simulink model "mrefrobotarm_modified_previous_y_error_previous_u"  (R2018b)
settings: Solver=FixedStepAuto  StartTime=0.0  StopTime=60  RelTol=1e-3  AbsTol=1e-6
undefined symbols (not defined in the file or in its folder): now, sfunxy2, simin
libraries: neural x368, simulink x1
(part 6 of 10)

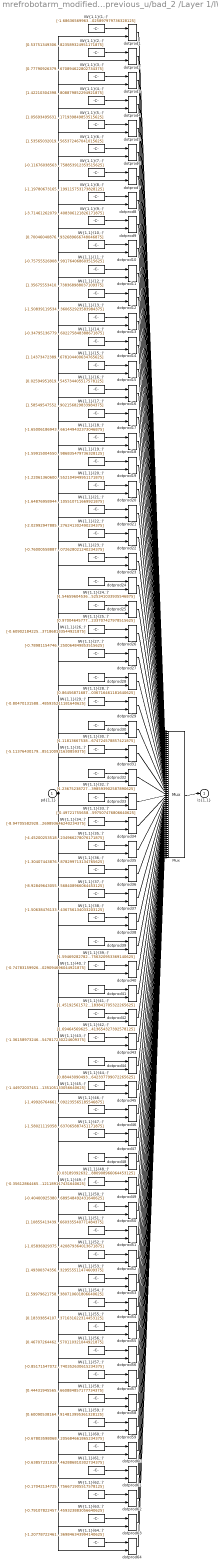
== system mrefrobotarm_modified_previous_y_error_previous_u/bad_2 /Layer 1/IW{1,1} ==
  "pd{1,1}" : Inport  PortDimensions=7
      mask Display: e = 0.06;c1 = [120 230 180]/255;c2 = ([120 230 180]+0)/(256+128);c3 = ([120 230 180]+128)/(256+128);patch([0 1 1 0],[0 0 1 1],c1);patch([0 1 1 1-e 1-e 0+e],[0 0 1 1-e 0+e 0+e],c2);patch([0 0 1 1-e 0+e 0+e],[0 1 1 1-e 1-e 0+e],c3);plot([0 1 1 0 0],[0 0 1 1 0]);
  "IW{1,1}(1,:)'" : Constant  Value=[-1.6863656996378744157283335880492813885211944580078125;-0.470597093744810790472143935403437353670597076416015625;0.381528307050592763172147670047706924378871917724609375;-1.12689962205123261895778341568075120449066162109375;-1.149898204806820256607124974834732711315155029296875;-1.0865193518723830212735492750653065741062164306640625;-0.6023983324376900316821092928876169025897979736328125]
      mask Display: e = 0.06;c1 = [120 150 230]/255;c2 = ([120 150 230]+0)/383;c3 = ([120 150 230]+128)/383;patch([0 1 1 0],[0 0 1 1],c1);patch([0 1 1 1-e 1-e 0+e],[0 0 1 1-e 0+e 0+e],c2);patch([0 0 1 1-e 0+e 0+e],[0 1 1 1-e 1-e 0+e],c3);plot([0 1 1 0 0],[0 0 1 1 0]);disp('Weights');
  "IW{1,1}(10,:)'" : Constant  Value=[0.70046040876794501972568696146481670439243316650390625;-0.59634747279149558085720173039590008556842803955078125;0.33402845316572282730049892052193172276020050048828125;-0.1546411702019059308810255970456637442111968994140625;1.35413836861219305518488909001462161540985107421875;1.7346283899615413393036078559816814959049224853515625;-0.56975117430301647214463400814565829932689666748046875]
      mask Display: e = 0.06;c1 = [120 150 230]/255;c2 = ([120 150 230]+0)/383;c3 = ([120 150 230]+128)/383;patch([0 1 1 0],[0 0 1 1],c1);patch([0 1 1 1-e 1-e 0+e],[0 0 1 1-e 0+e 0+e],c2);patch([0 0 1 1-e 0+e 0+e],[0 1 1 1-e 1-e 0+e],c3);plot([0 1 1 0 0],[0 0 1 1 0]);disp('Weights');
  "IW{1,1}(11,:)'" : Constant  Value=[-0.75755526908276149544718691686284728348255157470703125;-0.296579563589438433002243300506961531937122344970703125;0.497779535965763575422471376441535539925098419189453125;0.1665504115849312238850643552723340690135955810546875;-1.643932170348186172503801572020165622234344482421875;0.8794875708418334880889233318157494068145751953125;1.1526104705362014701819362016976810991764068603515625]
      mask Display: e = 0.06;c1 = [120 150 230]/255;c2 = ([120 150 230]+0)/383;c3 = ([120 150 230]+128)/383;patch([0 1 1 0],[0 0 1 1],c1);patch([0 1 1 1-e 1-e 0+e],[0 0 1 1-e 0+e 0+e],c2);patch([0 0 1 1-e 0+e 0+e],[0 1 1 1-e 1-e 0+e],c3);plot([0 1 1 0 0],[0 0 1 1 0]);disp('Weights');
  "IW{1,1}(12,:)'" : Constant  Value=[1.356755534102476179469931594212539494037628173828125;0.8249762999779475247663640402606688439846038818359375;0.11116932047618825751822413394620525650680065155029296875;-0.40444127320000544667522035524598322808742523193359375;-0.7395790815915237459421405219472944736480712890625;-1.102233156945345182720075172255747020244598388671875;1.5180689591781619807164815938449464738368988037109375]
      mask Display: e = 0.06;c1 = [120 150 230]/255;c2 = ([120 150 230]+0)/383;c3 = ([120 150 230]+128)/383;patch([0 1 1 0],[0 0 1 1],c1);patch([0 1 1 1-e 1-e 0+e],[0 0 1 1-e 0+e 0+e],c2);patch([0 0 1 1-e 0+e 0+e],[0 1 1 1-e 1-e 0+e],c3);plot([0 1 1 0 0],[0 0 1 1 0]);disp('Weights');
  "IW{1,1}(13,:)'" : Constant  Value=[-1.508391195342500878950886544771492481231689453125;0.1745384352813305894880357982401619665324687957763671875;-0.35046267193310509657777629399788565933704376220703125;0.70755991279883534428307712005334906280040740966796875;0.21164846614004406699649507572758011519908905029296875;3.394560192280937638287241497891955077648162841796875;2.8592038307015368303609648137353360652923583984375]
      mask Display: e = 0.06;c1 = [120 150 230]/255;c2 = ([120 150 230]+0)/383;c3 = ([120 150 230]+128)/383;patch([0 1 1 0],[0 0 1 1],c1);patch([0 1 1 1-e 1-e 0+e],[0 0 1 1-e 0+e 0+e],c2);patch([0 0 1 1-e 0+e 0+e],[0 1 1 1-e 1-e 0+e],c3);plot([0 1 1 0 0],[0 0 1 1 0]);disp('Weights');
  "IW{1,1}(14,:)'" : Constant  Value=[-0.347951367798633726113877173702348954975605010986328125;-1.1758278102151298316613292627152986824512481689453125;-1.4111353580198293666825293257716111838817596435546875;0.452708396797978529502159972253139130771160125732421875;0.57952339232880223374166916983085684478282928466796875;1.5762379928547864960108881859923712909221649169921875;0.9810342317283140545214337180368602275848388671875]
      mask Display: e = 0.06;c1 = [120 150 230]/255;c2 = ([120 150 230]+0)/383;c3 = ([120 150 230]+128)/383;patch([0 1 1 0],[0 0 1 1],c1);patch([0 1 1 1-e 1-e 0+e],[0 0 1 1-e 0+e 0+e],c2);patch([0 0 1 1-e 0+e 0+e],[0 1 1 1-e 1-e 0+e],c3);plot([0 1 1 0 0],[0 0 1 1 0]);disp('Weights');
  "IW{1,1}(15,:)'" : Constant  Value=[1.14373472389301156226792954839766025543212890625;0.9770289905242410810615183436311781406402587890625;-0.918973607377620016478658726555295288562774658203125;0.872028597290672724540172566776163876056671142578125;1.4709013012625096195051810354925692081451416015625;-0.1290434951660533735573466174173518083989620208740234375;0.66656798656280236148319318090216256678104400634765625]
      mask Display: e = 0.06;c1 = [120 150 230]/255;c2 = ([120 150 230]+0)/383;c3 = ([120 150 230]+128)/383;patch([0 1 1 0],[0 0 1 1],c1);patch([0 1 1 1-e 1-e 0+e],[0 0 1 1-e 0+e 0+e],c2);patch([0 0 1 1-e 0+e 0+e],[0 1 1 1-e 1-e 0+e],c3);plot([0 1 1 0 0],[0 0 1 1 0]);disp('Weights');
  "IW{1,1}(16,:)'" : Constant  Value=[0.025949518194994046493828676602788618765771389007568359375;1.056286903314246128360309739946387708187103271484375;1.3864161845839706455052464662003330886363983154296875;-0.62378102653036349156678852523327805101871490478515625;2.046193686105493458882165214163251221179962158203125;-0.0948604936613626492647455279438872821629047393798828125;1.4769159957528821269789887082879431545734405517578125]
      mask Display: e = 0.06;c1 = [120 150 230]/255;c2 = ([120 150 230]+0)/383;c3 = ([120 150 230]+128)/383;patch([0 1 1 0],[0 0 1 1],c1);patch([0 1 1 1-e 1-e 0+e],[0 0 1 1-e 0+e 0+e],c2);patch([0 0 1 1-e 0+e 0+e],[0 1 1 1-e 1-e 0+e],c3);plot([0 1 1 0 0],[0 0 1 1 0]);disp('Weights');
  "IW{1,1}(17,:)'" : Constant  Value=[1.5854954755240395769533279235474765300750732421875;0.062584963321976549988079341346747241914272308349609375;-1.086219183721052861102407405269332230091094970703125;-0.472400812961043137239158795637194998562335968017578125;-0.2084756610371170937323626048964797519147396087646484375;-1.2682346351539524054174989942112006247043609619140625;-2.59195409337992455078847342520020902156829833984375]
      mask Display: e = 0.06;c1 = [120 150 230]/255;c2 = ([120 150 230]+0)/383;c3 = ([120 150 230]+128)/383;patch([0 1 1 0],[0 0 1 1],c1);patch([0 1 1 1-e 1-e 0+e],[0 0 1 1-e 0+e 0+e],c2);patch([0 0 1 1-e 0+e 0+e],[0 1 1 1-e 1-e 0+e],c3);plot([0 1 1 0 0],[0 0 1 1 0]);disp('Weights');
  "IW{1,1}(18,:)'" : Constant  Value=[-1.6500618694364199701141160403494723141193389892578125;0.158471949334514750074021094405907206237316131591796875;1.605402587803847591629846647265367209911346435546875;-0.3344369037299077529468149805325083434581756591796875;0.357965741888847055474087710535968653857707977294921875;-2.016135923701856125234144201385788619518280029296875;-0.460005488291919728549572710107895545661449432373046875]
      mask Display: e = 0.06;c1 = [120 150 230]/255;c2 = ([120 150 230]+0)/383;c3 = ([120 150 230]+128)/383;patch([0 1 1 0],[0 0 1 1],c1);patch([0 1 1 1-e 1-e 0+e],[0 0 1 1-e 0+e 0+e],c2);patch([0 0 1 1-e 0+e 0+e],[0 1 1 1-e 1-e 0+e],c3);plot([0 1 1 0 0],[0 0 1 1 0]);disp('Weights');
  "IW{1,1}(19,:)'" : Constant  Value=[-1.5991500455075655651171473436988890171051025390625;1.348245600949198763629510722239501774311065673828125;0.80807469706489853944475498792598955333232879638671875;-1.7624762240675149183033454391988925635814666748046875;-1.016806479705910870592333594686351716518402099609375;0.300813059873307808711473398943780921399593353271484375;-1.634726680080462291044796074857003986835479736328125]
      mask Display: e = 0.06;c1 = [120 150 230]/255;c2 = ([120 150 230]+0)/383;c3 = ([120 150 230]+128)/383;patch([0 1 1 0],[0 0 1 1],c1);patch([0 1 1 1-e 1-e 0+e],[0 0 1 1-e 0+e 0+e],c2);patch([0 0 1 1-e 0+e 0+e],[0 1 1 1-e 1-e 0+e],c3);plot([0 1 1 0 0],[0 0 1 1 0]);disp('Weights');
  "IW{1,1}(2,:)'" : Constant  Value=[0.5375134930612259775983829968026839196681976318359375;-0.24811864763972335534703006487688980996608734130859375;-0.9050550568703263909497991335229016840457916259765625;-1.330177669034877663278848558547906577587127685546875;0.8445151037025706575178674029302783310413360595703125;0.453823539254982255553017012061900459229946136474609375;1.51432188940290313183822945575229823589324951171875]
      mask Display: e = 0.06;c1 = [120 150 230]/255;c2 = ([120 150 230]+0)/383;c3 = ([120 150 230]+128)/383;patch([0 1 1 0],[0 0 1 1],c1);patch([0 1 1 1-e 1-e 0+e],[0 0 1 1-e 0+e 0+e],c2);patch([0 0 1 1-e 0+e 0+e],[0 1 1 1-e 1-e 0+e],c3);plot([0 1 1 0 0],[0 0 1 1 0]);disp('Weights');
  "IW{1,1}(20,:)'" : Constant  Value=[-1.2206136060051242520074765707249753177165985107421875;1.2143694024926621199966803033021278679370880126953125;0.01284061424074450959154081175483952392823994159698486328125;0.674556463178389353885222590179182589054107666015625;0.82271266002563281372061965157627128064632415771484375;1.4603421023320530824918250800692476332187652587890625;-1.023340866984355113089577571372501552104949951171875]
      mask Display: e = 0.06;c1 = [120 150 230]/255;c2 = ([120 150 230]+0)/383;c3 = ([120 150 230]+128)/383;patch([0 1 1 0],[0 0 1 1],c1);patch([0 1 1 1-e 1-e 0+e],[0 0 1 1-e 0+e 0+e],c2);patch([0 0 1 1-e 0+e 0+e],[0 1 1 1-e 1-e 0+e],c3);plot([0 1 1 0 0],[0 0 1 1 0]);disp('Weights');
  "IW{1,1}(21,:)'" : Constant  Value=[-1.648769589442328875605880966759286820888519287109375;0.5674233186469184175848567974753677845001220703125;0.360630049005453423571765370070352219045162200927734375;0.72618846736561659671593815801315940916538238525390625;-1.6863477747584882937559314086684025824069976806640625;-0.543238509671011282620156634948216378688812255859375;-0.82507519282673491556323597251321189105510711669921875]
      mask Display: e = 0.06;c1 = [120 150 230]/255;c2 = ([120 150 230]+0)/383;c3 = ([120 150 230]+128)/383;patch([0 1 1 0],[0 0 1 1],c1);patch([0 1 1 1-e 1-e 0+e],[0 0 1 1-e 0+e 0+e],c2);patch([0 0 1 1-e 0+e 0+e],[0 1 1 1-e 1-e 0+e],c3);plot([0 1 1 0 0],[0 0 1 1 0]);disp('Weights');
  "IW{1,1}(22,:)'" : Constant  Value=[-2.02992947885647989636481725028716027736663818359375;-0.78930300349707904761231702650547958910465240478515625;-1.600745458741919424738853194867260754108428955078125;2.151514262201442040378651654464192688465118408203125;1.4383445102898109180245000970899127423763275146484375;1.0715968603907735090530195520841516554355621337890625;0.29850111989870364848087547215982340276241302490234375]
      mask Display: e = 0.06;c1 = [120 150 230]/255;c2 = ([120 150 230]+0)/383;c3 = ([120 150 230]+128)/383;patch([0 1 1 0],[0 0 1 1],c1);patch([0 1 1 1-e 1-e 0+e],[0 0 1 1-e 0+e 0+e],c2);patch([0 0 1 1-e 0+e 0+e],[0 1 1 1-e 1-e 0+e],c3);plot([0 1 1 0 0],[0 0 1 1 0]);disp('Weights');
  "IW{1,1}(23,:)'" : Constant  Value=[-0.7600055888729659869795796112157404422760009765625;0.71322247233798297116891262703575193881988525390625;1.917261913113857740853518407675437629222869873046875;0.056807101221510995781027730799905839376151561737060546875;0.6989265569105611586309123595128767192363739013671875;2.165339178672456288410330671467818319797515869140625;0.274757432287420166883151750880642794072628021240234375]
      mask Display: e = 0.06;c1 = [120 150 230]/255;c2 = ([120 150 230]+0)/383;c3 = ([120 150 230]+128)/383;patch([0 1 1 0],[0 0 1 1],c1);patch([0 1 1 1-e 1-e 0+e],[0 0 1 1-e 0+e 0+e],c2);patch([0 0 1 1-e 0+e 0+e],[0 1 1 1-e 1-e 0+e],c3);plot([0 1 1 0 0],[0 0 1 1 0]);disp('Weights');
  "IW{1,1}(24,:)'" : Constant  Value=[1.546596045364299509827787915128283202648162841796875;-1.8043253491178485869994574386510066688060760498046875;-1.0873028546852918641008045597118325531482696533203125;0.489548897640237345996183648821897804737091064453125;-1.0685662650111333871194574385299347341060638427734375;-2.01145955325918013301134124048985540866851806640625;-1.086944648018185244353617235901765525341033935546875]
      mask Display: e = 0.06;c1 = [120 150 230]/255;c2 = ([120 150 230]+0)/383;c3 = ([120 150 230]+128)/383;patch([0 1 1 0],[0 0 1 1],c1);patch([0 1 1 1-e 1-e 0+e],[0 0 1 1-e 0+e 0+e],c2);patch([0 0 1 1-e 0+e 0+e],[0 1 1 1-e 1-e 0+e],c3);plot([0 1 1 0 0],[0 0 1 1 0]);disp('Weights');
  "IW{1,1}(25,:)'" : Constant  Value=[0.97004645777546294471704868556116707623004913330078125;0.336271611140263881889467256769421510398387908935546875;0.2417062721643864764420328583582886494696140289306640625;1.4989475360339128418019072341849096119403839111328125;1.4380511250646048626578021867317147552967071533203125;1.1249383286835179518448057933710515499114990234375;0.2251758799012057166155642562443972565233707427978515625]
      mask Display: e = 0.06;c1 = [120 150 230]/255;c2 = ([120 150 230]+0)/383;c3 = ([120 150 230]+128)/383;patch([0 1 1 0],[0 0 1 1],c1);patch([0 1 1 1-e 1-e 0+e],[0 0 1 1-e 0+e 0+e],c2);patch([0 0 1 1-e 0+e 0+e],[0 1 1 1-e 1-e 0+e],c3);plot([0 1 1 0 0],[0 0 1 1 0]);disp('Weights');
  "IW{1,1}(26,:)'" : Constant  Value=[-0.60902184225669453443430256811552681028842926025390625;1.4626237168885207751145571819506585597991943359375;-0.283646747149560118916866713334457017481327056884765625;-0.41578668224785364504469953317311592400074005126953125;1.8146939194076010526401887545944191515445709228515625;-0.94831384411612063001228989378432743251323699951171875;0.99177285614588306383865301540936343371868133544921875]
      mask Display: e = 0.06;c1 = [120 150 230]/255;c2 = ([120 150 230]+0)/383;c3 = ([120 150 230]+128)/383;patch([0 1 1 0],[0 0 1 1],c1);patch([0 1 1 1-e 1-e 0+e],[0 0 1 1-e 0+e 0+e],c2);patch([0 0 1 1-e 0+e 0+e],[0 1 1 1-e 1-e 0+e],c3);plot([0 1 1 0 0],[0 0 1 1 0]);disp('Weights');
  "IW{1,1}(27,:)'" : Constant  Value=[-0.78981154746552861833919223499833606183528900146484375;-1.3508127899859114773306600909563712775707244873046875;0.4988288733380119577276445852476172149181365966796875;-0.761291513497599492410472521441988646984100341796875;1.513839332845589691345367100439034402370452880859375;1.038568147474759228998664184473454952239990234375;-1.2619104742456475065637278021313250064849853515625]
      mask Display: e = 0.06;c1 = [120 150 230]/255;c2 = ([120 150 230]+0)/383;c3 = ([120 150 230]+128)/383;patch([0 1 1 0],[0 0 1 1],c1);patch([0 1 1 1-e 1-e 0+e],[0 0 1 1-e 0+e 0+e],c2);patch([0 0 1 1-e 0+e 0+e],[0 1 1 1-e 1-e 0+e],c3);plot([0 1 1 0 0],[0 0 1 1 0]);disp('Weights');
  "IW{1,1}(28,:)'" : Constant  Value=[0.86456871687262815129315640660934150218963623046875;0.033660231342696848855222668817077646963298320770263671875;0.68849562687325371879154545240453444421291351318359375;1.05512528935876037650132275302894413471221923828125;1.3310343837191738192160528342355974018573760986328125;1.4214566142145310667643798296921886503696441650390625;-0.91698163671545673825136191226192750036716461181640625]
      mask Display: e = 0.06;c1 = [120 150 230]/255;c2 = ([120 150 230]+0)/383;c3 = ([120 150 230]+128)/383;patch([0 1 1 0],[0 0 1 1],c1);patch([0 1 1 1-e 1-e 0+e],[0 0 1 1-e 0+e 0+e],c2);patch([0 0 1 1-e 0+e 0+e],[0 1 1 1-e 1-e 0+e],c3);plot([0 1 1 0 0],[0 0 1 1 0]);disp('Weights');
  "IW{1,1}(29,:)'" : Constant  Value=[-0.80470131588495730223797863800427876412868499755859375;-1.6155846603753911683298838397604413330554962158203125;-0.29114476463801874928094548522494733333587646484375;0.75042474844354678520375045991386286914348602294921875;1.7495307116501146449394354931428097188472747802734375;-0.3413257555915460983442244469188153743743896484375;-0.382665686428625806403402975774952210485935211181640625]
      mask Display: e = 0.06;c1 = [120 150 230]/255;c2 = ([120 150 230]+0)/383;c3 = ([120 150 230]+128)/383;patch([0 1 1 0],[0 0 1 1],c1);patch([0 1 1 1-e 1-e 0+e],[0 0 1 1-e 0+e 0+e],c2);patch([0 0 1 1-e 0+e 0+e],[0 1 1 1-e 1-e 0+e],c3);plot([0 1 1 0 0],[0 0 1 1 0]);disp('Weights');
  "IW{1,1}(3,:)'" : Constant  Value=[0.77790926379179115013329237626749090850353240966796875;1.597997887025701668761712426203303039073944091796875;-0.061513463120482343715611506240747985430061817169189453125;0.7694262824388911070627727895043790340423583984375;0.53571795086796225593417375421267934143543243408203125;1.255108578389512619111201274790801107883453369140625;-1.12287357758761885406784131191670894622802734375]
      mask Display: e = 0.06;c1 = [120 150 230]/255;c2 = ([120 150 230]+0)/383;c3 = ([120 150 230]+128)/383;patch([0 1 1 0],[0 0 1 1],c1);patch([0 1 1 1-e 1-e 0+e],[0 0 1 1-e 0+e 0+e],c2);patch([0 0 1 1-e 0+e 0+e],[0 1 1 1-e 1-e 0+e],c3);plot([0 1 1 0 0],[0 0 1 1 0]);disp('Weights');
  "IW{1,1}(30,:)'" : Constant  Value=[1.11813667538101402243455595453269779682159423828125;-2.0011147436250649178646199288778007030487060546875;-1.2389603095632202300890867263660766184329986572265625;0.99632266524748314129311665965360589325428009033203125;-0.1464403285517131558801651181056513451039791107177734375;1.78125755432936383471087538055144250392913818359375;1.7380547403563877395527015323750674724578857421875]
      mask Display: e = 0.06;c1 = [120 150 230]/255;c2 = ([120 150 230]+0)/383;c3 = ([120 150 230]+128)/383;patch([0 1 1 0],[0 0 1 1],c1);patch([0 1 1 1-e 1-e 0+e],[0 0 1 1-e 0+e 0+e],c2);patch([0 0 1 1-e 0+e 0+e],[0 1 1 1-e 1-e 0+e],c3);plot([0 1 1 0 0],[0 0 1 1 0]);disp('Weights');
  "IW{1,1}(31,:)'" : Constant  Value=[-5.1137643017961860181230804300867021083831787109375;1.3370606083956821930058822545106522738933563232421875;2.442518793233874330184107748209498822689056396484375;0.6028625806456482383310913064633496105670928955078125;-1.92576905446539026200980515568517148494720458984375;-0.6757333917518464350138174268067814409732818603515625;0.81038330323658624987359644364914856851100921630859375]
      mask Display: e = 0.06;c1 = [120 150 230]/255;c2 = ([120 150 230]+0)/383;c3 = ([120 150 230]+128)/383;patch([0 1 1 0],[0 0 1 1],c1);patch([0 1 1 1-e 1-e 0+e],[0 0 1 1-e 0+e 0+e],c2);patch([0 0 1 1-e 0+e 0+e],[0 1 1 1-e 1-e 0+e],c3);plot([0 1 1 0 0],[0 0 1 1 0]);disp('Weights');
  "IW{1,1}(32,:)'" : Constant  Value=[1.2367523872787222760649683550582267343997955322265625;-0.784854563913853997547676044632680714130401611328125;-1.439473545848857671813902925350703299045562744140625;1.09236546200067241585429655970074236392974853515625;1.0496288292411153353356212392100133001804351806640625;0.06836094254987955254332376853199093602597713470458984375;-1.286462130941723902566309334360994398593902587890625]
      mask Display: e = 0.06;c1 = [120 150 230]/255;c2 = ([120 150 230]+0)/383;c3 = ([120 150 230]+128)/383;patch([0 1 1 0],[0 0 1 1],c1);patch([0 1 1 1-e 1-e 0+e],[0 0 1 1-e 0+e 0+e],c2);patch([0 0 1 1-e 0+e 0+e],[0 1 1 1-e 1-e 0+e],c3);plot([0 1 1 0 0],[0 0 1 1 0]);disp('Weights');
  "IW{1,1}(33,:)'" : Constant  Value=[-0.4972175565835499355671345256268978118896484375;1.01628497643774817760231599095277488231658935546875;1.705775427614244943441690338659100234508514404296875;-0.155163647387632275265190173740847967565059661865234375;-0.38711282558761184180440295676817186176776885986328125;0.6706206203731606141360543915652669966220855712890625;-1.11530850752759480570830419310368597507476806640625]
      mask Display: e = 0.06;c1 = [120 150 230]/255;c2 = ([120 150 230]+0)/383;c3 = ([120 150 230]+128)/383;patch([0 1 1 0],[0 0 1 1],c1);patch([0 1 1 1-e 1-e 0+e],[0 0 1 1-e 0+e 0+e],c2);patch([0 0 1 1-e 0+e 0+e],[0 1 1 1-e 1-e 0+e],c3);plot([0 1 1 0 0],[0 0 1 1 0]);disp('Weights');
  "IW{1,1}(34,:)'" : Constant  Value=[-8.9470558292806234845784274511970579624176025390625;5.86025071287466925440412524039857089519500732421875;0.89003059289749819615877868272946216166019439697265625;-0.006319623623432799215671185066867110435850918292999267578125;1.1887800724449284484052213883842341601848602294921875;3.9517133987949062401412447798065841197967529296875;2.4410282631594579783040899201296269893646240234375]
      mask Display: e = 0.06;c1 = [120 150 230]/255;c2 = ([120 150 230]+0)/383;c3 = ([120 150 230]+128)/383;patch([0 1 1 0],[0 0 1 1],c1);patch([0 1 1 1-e 1-e 0+e],[0 0 1 1-e 0+e 0+e],c2);patch([0 0 1 1-e 0+e 0+e],[0 1 1 1-e 1-e 0+e],c3);plot([0 1 1 0 0],[0 0 1 1 0]);disp('Weights');
  "IW{1,1}(35,:)'" : Constant  Value=[-4.45200253518322863754974605399183928966522216796875;1.0956730899398532397270855653914622962474822998046875;-0.296116424887555407252648365101777017116546630859375;1.494172243435615943241145942010916769504547119140625;-1.405105462929962190088417628430761396884918212890625;-1.8065586582246557778574924668646417558193206787109375;-2.091504311274504868123358392040245234966278076171875]
      mask Display: e = 0.06;c1 = [120 150 230]/255;c2 = ([120 150 230]+0)/383;c3 = ([120 150 230]+128)/383;patch([0 1 1 0],[0 0 1 1],c1);patch([0 1 1 1-e 1-e 0+e],[0 0 1 1-e 0+e 0+e],c2);patch([0 0 1 1-e 0+e 0+e],[0 1 1 1-e 1-e 0+e],c3);plot([0 1 1 0 0],[0 0 1 1 0]);disp('Weights');
  "IW{1,1}(36,:)'" : Constant  Value=[-1.3040744387684621852230293370666913688182830810546875;-1.0839533773058225296637147039291448891162872314453125;1.1996912135972817026186021394096314907073974609375;0.299632799474621902557913699638447724282741546630859375;-1.0338437717971202811639841456781141459941864013671875;1.060633860379795123662916012108325958251953125;0.80119404908470548409837874714867211878299713134765625]
      mask Display: e = 0.06;c1 = [120 150 230]/255;c2 = ([120 150 230]+0)/383;c3 = ([120 150 230]+128)/383;patch([0 1 1 0],[0 0 1 1],c1);patch([0 1 1 1-e 1-e 0+e],[0 0 1 1-e 0+e 0+e],c2);patch([0 0 1 1-e 0+e 0+e],[0 1 1 1-e 1-e 0+e],c3);plot([0 1 1 0 0],[0 0 1 1 0]);disp('Weights');
  "IW{1,1}(37,:)'" : Constant  Value=[-8.928496430556503327125028590671718120574951171875;6.41281098021677653520100648165680468082427978515625;1.292318686852158560185444002854637801647186279296875;-1.0169657309557076363404348740004934370517730712890625;-1.4447233934709735603263425218756310641765594482421875;-1.8212597060116382241545807119109667837619781494140625;-2.000066902793254275394474461791105568408966064453125]
      mask Display: e = 0.06;c1 = [120 150 230]/255;c2 = ([120 150 230]+0)/383;c3 = ([120 150 230]+128)/383;patch([0 1 1 0],[0 0 1 1],c1);patch([0 1 1 1-e 1-e 0+e],[0 0 1 1-e 0+e 0+e],c2);patch([0 0 1 1-e 0+e 0+e],[0 1 1 1-e 1-e 0+e],c3);plot([0 1 1 0 0],[0 0 1 1 0]);disp('Weights');
  "IW{1,1}(38,:)'" : Constant  Value=[-1.5063847613337173481085073944996111094951629638671875;-0.92097648878295623742218367624445818364620208740234375;-0.9838165288434570499020992428995668888092041015625;-0.33928758212320830889296985333203338086605072021484375;-0.60176867956408575111026948434300720691680908203125;0.52167233477996066692838894596206955611705780029296875;-0.901664409713287984260432494920678436756134033203125]
      mask Display: e = 0.06;c1 = [120 150 230]/255;c2 = ([120 150 230]+0)/383;c3 = ([120 150 230]+128)/383;patch([0 1 1 0],[0 0 1 1],c1);patch([0 1 1 1-e 1-e 0+e],[0 0 1 1-e 0+e 0+e],c2);patch([0 0 1 1-e 0+e 0+e],[0 1 1 1-e 1-e 0+e],c3);plot([0 1 1 0 0],[0 0 1 1 0]);disp('Weights');
  "IW{1,1}(39,:)'" : Constant  Value=[1.594692827829733428046665721922181546688079833984375;-0.431588743177177491805451836626161821186542510986328125;-0.5767038172813823138085354003123939037322998046875;-1.4856881211963273159426535130478441715240478515625;-1.537250986312717504489455677685327827930450439453125;-1.5160546591084627099377257763990201056003570556640625;0.02677171951358392476549852290190756320953369140625]
      mask Display: e = 0.06;c1 = [120 150 230]/255;c2 = ([120 150 230]+0)/383;c3 = ([120 150 230]+128)/383;patch([0 1 1 0],[0 0 1 1],c1);patch([0 1 1 1-e 1-e 0+e],[0 0 1 1-e 0+e 0+e],c2);patch([0 0 1 1-e 0+e 0+e],[0 1 1 1-e 1-e 0+e],c3);plot([0 1 1 0 0],[0 0 1 1 0]);disp('Weights');
  "IW{1,1}(4,:)'" : Constant  Value=[1.4221030439802160305617917401832528412342071533203125;-0.719802079075858358692130423150956630706787109375;0.390203414206296839150667210560641251504421234130859375;-1.40290775448764382105082404450513422489166259765625;-0.246566272133671715582892147722304798662662506103515625;0.978533484262781971807498848647810518741607666015625;0.72315047260570686216141211843932978808879852294921875]
      mask Display: e = 0.06;c1 = [120 150 230]/255;c2 = ([120 150 230]+0)/383;c3 = ([120 150 230]+128)/383;patch([0 1 1 0],[0 0 1 1],c1);patch([0 1 1 1-e 1-e 0+e],[0 0 1 1-e 0+e 0+e],c2);patch([0 0 1 1-e 0+e 0+e],[0 1 1 1-e 1-e 0+e],c3);plot([0 1 1 0 0],[0 0 1 1 0]);disp('Weights');
  "IW{1,1}(40,:)'" : Constant  Value=[-0.74783159926091802294223498392966575920581817626953125;-0.0156016786915698472959501685863870079629123210906982421875;1.205674453621349950793728567077778279781341552734375;-0.642379166939826884430431164219044148921966552734375;-2.3466396920997372177453144104219973087310791015625;2.003758055175307806194950899225659668445587158203125;0.457948677082519572945074060044134967029094696044921875]
      mask Display: e = 0.06;c1 = [120 150 230]/255;c2 = ([120 150 230]+0)/383;c3 = ([120 150 230]+128)/383;patch([0 1 1 0],[0 0 1 1],c1);patch([0 1 1 1-e 1-e 0+e],[0 0 1 1-e 0+e 0+e],c2);patch([0 0 1 1-e 0+e 0+e],[0 1 1 1-e 1-e 0+e],c3);plot([0 1 1 0 0],[0 0 1 1 0]);disp('Weights');
  "IW{1,1}(41,:)'" : Constant  Value=[1.451925615721403328706173851969651877880096435546875;0.893887593572912475536895726691000163555145263671875;-0.47449044571051024465901946314261294901371002197265625;-1.1508731751823262356992927379906177520751953125;-0.45410349609860478636846892186440527439117431640625;0.194166359333692917221725338094984181225299835205078125;-1.4499390721543312654517876580939628183841705322265625]
      mask Display: e = 0.06;c1 = [120 150 230]/255;c2 = ([120 150 230]+0)/383;c3 = ([120 150 230]+128)/383;patch([0 1 1 0],[0 0 1 1],c1);patch([0 1 1 1-e 1-e 0+e],[0 0 1 1-e 0+e 0+e],c2);patch([0 0 1 1-e 0+e 0+e],[0 1 1 1-e 1-e 0+e],c3);plot([0 1 1 0 0],[0 0 1 1 0]);disp('Weights');
  "IW{1,1}(42,:)'" : Constant  Value=[1.6946456962588474226549806189723312854766845703125;0.425834425212213874001321300966083072125911712646484375;-0.12820727712798618558309726722654886543750762939453125;0.82693407426810916494019920719438232481479644775390625;-0.686592815915464171894200262613594532012939453125;-1.758457794378568639359627923113293945789337158203125;-1.16195091792224758364682202227413654327392578125]
      mask Display: e = 0.06;c1 = [120 150 230]/255;c2 = ([120 150 230]+0)/383;c3 = ([120 150 230]+128)/383;patch([0 1 1 0],[0 0 1 1],c1);patch([0 1 1 1-e 1-e 0+e],[0 0 1 1-e 0+e 0+e],c2);patch([0 0 1 1-e 0+e 0+e],[0 1 1 1-e 1-e 0+e],c3);plot([0 1 1 0 0],[0 0 1 1 0]);disp('Weights');
  "IW{1,1}(43,:)'" : Constant  Value=[-1.3615897324638819299025271902792155742645263671875;0.278290236737857521465144827743642963469028472900390625;-1.0667263436467611104063735183444805443286895751953125;0.5094403583366851062663727134349755942821502685546875;-0.3608847114676769773922160311485640704631805419921875;-1.6444246535543662890432869971846230328083038330078125;0.2014908543440262211898783561991876922547817230224609375]
      mask Display: e = 0.06;c1 = [120 150 230]/255;c2 = ([120 150 230]+0)/383;c3 = ([120 150 230]+128)/383;patch([0 1 1 0],[0 0 1 1],c1);patch([0 1 1 1-e 1-e 0+e],[0 0 1 1-e 0+e 0+e],c2);patch([0 0 1 1-e 0+e 0+e],[0 1 1 1-e 1-e 0+e],c3);plot([0 1 1 0 0],[0 0 1 1 0]);disp('Weights');
  "IW{1,1}(44,:)'" : Constant  Value=[0.88443090493589926470718864948139525949954986572265625;-0.85802238734703450973029248416423797607421875;1.324391165572524453608593830722384154796600341796875;0.461782793456212814486860906981746666133403778076171875;1.661385307581995096626314989407546818256378173828125;0.945152587292386936468346902984194457530975341796875;-0.9266743481198551624089532197103835642337799072265625]
      mask Display: e = 0.06;c1 = [120 150 230]/255;c2 = ([120 150 230]+0)/383;c3 = ([120 150 230]+128)/383;patch([0 1 1 0],[0 0 1 1],c1);patch([0 1 1 1-e 1-e 0+e],[0 0 1 1-e 0+e 0+e],c2);patch([0 0 1 1-e 0+e 0+e],[0 1 1 1-e 1-e 0+e],c3);plot([0 1 1 0 0],[0 0 1 1 0]);disp('Weights');
  "IW{1,1}(45,:)'" : Constant  Value=[-1.4497203745100188942984686946147121489048004150390625;-1.0724545486426311224903429319965653121471405029296875;-0.1484734504477010219591903705804725177586078643798828125;1.16702814752873873516136882244609296321868896484375;-0.2635918282285700797729077748954296112060546875;0.425653140911482708030888488792697899043560028076171875;-1.2814010493250835853729086011298932135105133056640625]
      mask Display: e = 0.06;c1 = [120 150 230]/255;c2 = ([120 150 230]+0)/383;c3 = ([120 150 230]+128)/383;patch([0 1 1 0],[0 0 1 1],c1);patch([0 1 1 1-e 1-e 0+e],[0 0 1 1-e 0+e 0+e],c2);patch([0 0 1 1-e 0+e 0+e],[0 1 1 1-e 1-e 0+e],c3);plot([0 1 1 0 0],[0 0 1 1 0]);disp('Weights');
  "IW{1,1}(46,:)'" : Constant  Value=[-1.499267646611195825556706040515564382076263427734375;1.3174488089667761858692074383725412189960479736328125;-0.5399640277496706719517760575399734079837799072265625;0.74937954858944155756006466617691330611705780029296875;0.827336789688755569471823037019930779933929443359375;0.69217529344171391247897417997592128813266754150390625;-0.0098935374971492288931340652879953267984092235565185546875]
      mask Display: e = 0.06;c1 = [120 150 230]/255;c2 = ([120 150 230]+0)/383;c3 = ([120 150 230]+128)/383;patch([0 1 1 0],[0 0 1 1],c1);patch([0 1 1 1-e 1-e 0+e],[0 0 1 1-e 0+e 0+e],c2);patch([0 0 1 1-e 0+e 0+e],[0 1 1 1-e 1-e 0+e],c3);plot([0 1 1 0 0],[0 0 1 1 0]);disp('Weights');
  "IW{1,1}(47,:)'" : Constant  Value=[-1.580211193585773887804180048988200724124908447265625;2.390564368106120607393449972732923924922943115234375;1.6877873845365360949699606862850487232208251953125;-1.2944633535895053721986869277316145598888397216796875;-1.7480708568408029890406396589241921901702880859375;-1.3227414561588266561642512897378765046596527099609375;0.0080150553368121095487719429684148053638637065887451171875]
      mask Display: e = 0.06;c1 = [120 150 230]/255;c2 = ([120 150 230]+0)/383;c3 = ([120 150 230]+128)/383;patch([0 1 1 0],[0 0 1 1],c1);patch([0 1 1 1-e 1-e 0+e],[0 0 1 1-e 0+e 0+e],c2);patch([0 0 1 1-e 0+e 0+e],[0 1 1 1-e 1-e 0+e],c3);plot([0 1 1 0 0],[0 0 1 1 0]);disp('Weights');
  "IW{1,1}(48,:)'" : Constant  Value=[0.031893926326842854390708481560068321414291858673095703125;0.70069625805801416529305924996151588857173919677734375;0.049271889340007597735127120586184901185333728790283203125;-0.74807700353605144361068823855021037161350250244140625;-1.6080986723792289883050443677348084747791290283203125;2.6854530240896803405803439090959727764129638671875;1.0569473231406949498278891041991300880908966064453125]
      mask Display: e = 0.06;c1 = [120 150 230]/255;c2 = ([120 150 230]+0)/383;c3 = ([120 150 230]+128)/383;patch([0 1 1 0],[0 0 1 1],c1);patch([0 1 1 1-e 1-e 0+e],[0 0 1 1-e 0+e 0+e],c2);patch([0 0 1 1-e 0+e 0+e],[0 1 1 1-e 1-e 0+e],c3);plot([0 1 1 0 0],[0 0 1 1 0]);disp('Weights');
  "IW{1,1}(49,:)'" : Constant  Value=[-0.35612864465414595382952711588586680591106414794921875;1.9304518881102905591973240007064305245876312255859375;-0.9617104874235191669384903434547595679759979248046875;1.1702147778362237406923895832733251154422760009765625;-0.4409392174295903021885578709770925343036651611328125;-0.38543466310173968292218660280923359096050262451171875;-0.61003965689040173803192601553746499121189117431640625]
      mask Display: e = 0.06;c1 = [120 150 230]/255;c2 = ([120 150 230]+0)/383;c3 = ([120 150 230]+128)/383;patch([0 1 1 0],[0 0 1 1],c1);patch([0 1 1 1-e 1-e 0+e],[0 0 1 1-e 0+e 0+e],c2);patch([0 0 1 1-e 0+e 0+e],[0 1 1 1-e 1-e 0+e],c3);plot([0 1 1 0 0],[0 0 1 1 0]);disp('Weights');
  "IW{1,1}(5,:)'" : Constant  Value=[1.05693495631027278847113848314620554447174072265625;-0.91310152750909578944771283204318024218082427978515625;1.2156917518958338941814645295380614697933197021484375;0.46715729048266985135029472075984813272953033447265625;0.7054023909970232875110696113551966845989227294921875;-1.2605475334731870429294531277264468371868133544921875;-0.67153241564735266511121380972326733171939849853515625]
      mask Display: e = 0.06;c1 = [120 150 230]/255;c2 = ([120 150 230]+0)/383;c3 = ([120 150 230]+128)/383;patch([0 1 1 0],[0 0 1 1],c1);patch([0 1 1 1-e 1-e 0+e],[0 0 1 1-e 0+e 0+e],c2);patch([0 0 1 1-e 0+e 0+e],[0 1 1 1-e 1-e 0+e],c3);plot([0 1 1 0 0],[0 0 1 1 0]);disp('Weights');
  "IW{1,1}(50,:)'" : Constant  Value=[-0.404009253806436208211749772090115584433078765869140625;-1.2315947097517219166462609791778959333896636962890625;-1.4211961443024956341929510017507709562778472900390625;-0.8014760631940216484281336306594312191009521484375;0.38100646019661887908824837722931988537311553955078125;-1.6770917838081056405741264825337566435337066650390625;-1.1452718916317794484172054580994881689548492431640625]
      mask Display: e = 0.06;c1 = [120 150 230]/255;c2 = ([120 150 230]+0)/383;c3 = ([120 150 230]+128)/383;patch([0 1 1 0],[0 0 1 1],c1);patch([0 1 1 1-e 1-e 0+e],[0 0 1 1-e 0+e 0+e],c2);patch([0 0 1 1-e 0+e 0+e],[0 1 1 1-e 1-e 0+e],c3);plot([0 1 1 0 0],[0 0 1 1 0]);disp('Weights');
  "IW{1,1}(51,:)'" : Constant  Value=[1.1085541343952647341808415148989297449588775634765625;-0.07407285789749377957758014190403628163039684295654296875;-0.9065560472035958383685283479280769824981689453125;1.3602585164200260425815258713555522263050079345703125;-0.963885894612861005015247428673319518566131591796875;1.4465559289898430872511880806996487081050872802734375;-0.027960827926225194361986581270684837363660335540771484375]
      mask Display: e = 0.06;c1 = [120 150 230]/255;c2 = ([120 150 230]+0)/383;c3 = ([120 150 230]+128)/383;patch([0 1 1 0],[0 0 1 1],c1);patch([0 1 1 1-e 1-e 0+e],[0 0 1 1-e 0+e 0+e],c2);patch([0 0 1 1-e 0+e 0+e],[0 1 1 1-e 1-e 0+e],c3);plot([0 1 1 0 0],[0 0 1 1 0]);disp('Weights');
  "IW{1,1}(52,:)'" : Constant  Value=[-1.0583692937576234527341512148268520832061767578125;-1.8322459544312652557351839277544058859348297119140625;1.5074415180687783522017753057298250496387481689453125;-0.73959332194639426649729330165428109467029571533203125;0.937981466166692978703167682397179305553436279296875;-0.903262305677095422851152761722914874553680419921875;0.351679789348338101007129807840101420879364013671875]
      mask Display: e = 0.06;c1 = [120 150 230]/255;c2 = ([120 150 230]+0)/383;c3 = ([120 150 230]+128)/383;patch([0 1 1 0],[0 0 1 1],c1);patch([0 1 1 1-e 1-e 0+e],[0 0 1 1-e 0+e 0+e],c2);patch([0 0 1 1-e 0+e 0+e],[0 1 1 1-e 1-e 0+e],c3);plot([0 1 1 0 0],[0 0 1 1 0]);disp('Weights');
  "IW{1,1}(53,:)'" : Constant  Value=[1.493003743566507779405583278276026248931884765625;1.040494323473815985181545329396612942218780517578125;1.6685042581210429712967879822826944291591644287109375;-0.1267792601195900370480984520327183417975902557373046875;-1.3199548235819802410873080589226447045803070068359375;-0.83687794665296910689988862941390834748744964599609375;-0.05751615341538494907691614344003028236329555511474609375]
      mask Display: e = 0.06;c1 = [120 150 230]/255;c2 = ([120 150 230]+0)/383;c3 = ([120 150 230]+128)/383;patch([0 1 1 0],[0 0 1 1],c1);patch([0 1 1 1-e 1-e 0+e],[0 0 1 1-e 0+e 0+e],c2);patch([0 0 1 1-e 0+e 0+e],[0 1 1 1-e 1-e 0+e],c3);plot([0 1 1 0 0],[0 0 1 1 0]);disp('Weights');
  "IW{1,1}(54,:)'" : Constant  Value=[1.5997962175819739893967152966069988906383514404296875;-1.3240704130395404281017590619740076363086700439453125;0.43843418447456283804086751842987723648548126220703125;0.29941738624136682300758138808305375277996063232421875;1.12194245825770710922597572789527475833892822265625;-0.131693466742203668662369864250649698078632354736328125;0.77083193753003487191932663336046971380710601806640625]
      mask Display: e = 0.06;c1 = [120 150 230]/255;c2 = ([120 150 230]+0)/383;c3 = ([120 150 230]+128)/383;patch([0 1 1 0],[0 0 1 1],c1);patch([0 1 1 1-e 1-e 0+e],[0 0 1 1-e 0+e 0+e],c2);patch([0 0 1 1-e 0+e 0+e],[0 1 1 1-e 1-e 0+e],c3);plot([0 1 1 0 0],[0 0 1 1 0]);disp('Weights');
  "IW{1,1}(55,:)'" : Constant  Value=[0.18333854107646063713588091559358872473239898681640625;0.61476214805657836137697813683189451694488525390625;1.053931311637554824045537316123954951763153076171875;-0.26875543923902178722329381344025023281574249267578125;-1.902654712044029139406120521016418933868408203125;-1.09195876341819886334860711940564215183258056640625;0.315464766408472929715145482987281866371631622314453125]
      mask Display: e = 0.06;c1 = [120 150 230]/255;c2 = ([120 150 230]+0)/383;c3 = ([120 150 230]+128)/383;patch([0 1 1 0],[0 0 1 1],c1);patch([0 1 1 1-e 1-e 0+e],[0 0 1 1-e 0+e 0+e],c2);patch([0 0 1 1-e 0+e 0+e],[0 1 1 1-e 1-e 0+e],c3);plot([0 1 1 0 0],[0 0 1 1 0]);disp('Weights');
  "IW{1,1}(56,:)'" : Constant  Value=[0.4670726446264883424674962952849455177783966064453125;-0.84659853182582989195026357265305705368518829345703125;-0.34927575690305712186045639100484549999237060546875;-0.75239684609279333660225574931246228516101837158203125;-1.147014630769624066175538246170617640018463134765625;1.4354243192586386701492529027746059000492095947265625;1.133136993498858213769153735483996570110321044921875]
      mask Display: e = 0.06;c1 = [120 150 230]/255;c2 = ([120 150 230]+0)/383;c3 = ([120 150 230]+128)/383;patch([0 1 1 0],[0 0 1 1],c1);patch([0 1 1 1-e 1-e 0+e],[0 0 1 1-e 0+e 0+e],c2);patch([0 0 1 1-e 0+e 0+e],[0 1 1 1-e 1-e 0+e],c3);plot([0 1 1 0 0],[0 0 1 1 0]);disp('Weights');
  "IW{1,1}(57,:)'" : Constant  Value=[-0.85171547072790987353840819196193479001522064208984375;0.425745603454170284951629810166195966303348541259765625;-1.2662287700325995931649458725587464869022369384765625;-1.0407026433754318350821677086059935390949249267578125;1.2629609214528649818731764753465540707111358642578125;-0.10416975369531868145234199118931428529322147369384765625;1.05206010681049999533342997892759740352630615234375]
      mask Display: e = 0.06;c1 = [120 150 230]/255;c2 = ([120 150 230]+0)/383;c3 = ([120 150 230]+128)/383;patch([0 1 1 0],[0 0 1 1],c1);patch([0 1 1 1-e 1-e 0+e],[0 0 1 1-e 0+e 0+e],c2);patch([0 0 1 1-e 0+e 0+e],[0 1 1 1-e 1-e 0+e],c3);plot([0 1 1 0 0],[0 0 1 1 0]);disp('Weights');
  "IW{1,1}(58,:)'" : Constant  Value=[0.444319455656049189240519581289845518767833709716796875;0.6265749100594339981995517518953420221805572509765625;0.9397420640044160666803918502409942448139190673828125;-1.2777767800898207628534919422236271202564239501953125;-1.06186091573441832025537223671562969684600830078125;-0.77288868311795388965634856504038907587528228759765625;1.2593236317262659351712272837175987660884857177734375]
      mask Display: e = 0.06;c1 = [120 150 230]/255;c2 = ([120 150 230]+0)/383;c3 = ([120 150 230]+128)/383;patch([0 1 1 0],[0 0 1 1],c1);patch([0 1 1 1-e 1-e 0+e],[0 0 1 1-e 0+e 0+e],c2);patch([0 0 1 1-e 0+e 0+e],[0 1 1 1-e 1-e 0+e],c3);plot([0 1 1 0 0],[0 0 1 1 0]);disp('Weights');
  "IW{1,1}(59,:)'" : Constant  Value=[0.6009053816497498257120923881302587687969207763671875;0.308150927658255413543741951798438094556331634521484375;-1.40244011299734072650835514650680124759674072265625;-1.0193265064390828467111305144499056041240692138671875;-0.383269137858561759202302710036747157573699951171875;-1.9544121939296559276044717989861965179443359375;-0.66119992097470714487172926965286023914813995361328125]
      mask Display: e = 0.06;c1 = [120 150 230]/255;c2 = ([120 150 230]+0)/383;c3 = ([120 150 230]+128)/383;patch([0 1 1 0],[0 0 1 1],c1);patch([0 1 1 1-e 1-e 0+e],[0 0 1 1-e 0+e 0+e],c2);patch([0 0 1 1-e 0+e 0+e],[0 1 1 1-e 1-e 0+e],c3);plot([0 1 1 0 0],[0 0 1 1 0]);disp('Weights');
  "IW{1,1}(6,:)'" : Constant  Value=[1.535650320196232154756899035419337451457977294921875;1.16959402883453567056903921184130012989044189453125;-0.60943990596203356790994121183757670223712921142578125;-0.318550588995249406298881922339205630123615264892578125;1.432218515173481865332405504886992275714874267578125;0.61686536373397948818109171043033711612224578857421875;0.489942496690119411173469643472344614565372467041015625]
      mask Display: e = 0.06;c1 = [120 150 230]/255;c2 = ([120 150 230]+0)/383;c3 = ([120 150 230]+128)/383;patch([0 1 1 0],[0 0 1 1],c1);patch([0 1 1 1-e 1-e 0+e],[0 0 1 1-e 0+e 0+e],c2);patch([0 0 1 1-e 0+e 0+e],[0 1 1 1-e 1-e 0+e],c3);plot([0 1 1 0 0],[0 0 1 1 0]);disp('Weights');
  "IW{1,1}(60,:)'" : Constant  Value=[-0.67803598068871784310118755456642247736454010009765625;1.3523214381693391406003001975477673113346099853515625;1.3965897080101579152966451147221960127353668212890625;1.0263464080657056509693347834399901330471038818359375;-0.10053769535427738157640220606481307186186313629150390625;-0.10147476457780069125647059991024434566497802734375;1.0341403343742834319840540047152899205684661865234375]
      mask Display: e = 0.06;c1 = [120 150 230]/255;c2 = ([120 150 230]+0)/383;c3 = ([120 150 230]+128)/383;patch([0 1 1 0],[0 0 1 1],c1);patch([0 1 1 1-e 1-e 0+e],[0 0 1 1-e 0+e 0+e],c2);patch([0 0 1 1-e 0+e 0+e],[0 1 1 1-e 1-e 0+e],c3);plot([0 1 1 0 0],[0 0 1 1 0]);disp('Weights');
  "IW{1,1}(61,:)'" : Constant  Value=[-0.63857231918558243766170789967873133718967437744140625;0.98455177052132236692472133654518984258174896240234375;-1.24228157194427790699364777537994086742401123046875;-0.35251749058152892501993846963159739971160888671875;-0.410375404744263760914435579252312891185283660888671875;-1.1850465837103227872972865952760912477970123291015625;-1.256024188662047347264660857035778462886810302734375]
      mask Display: e = 0.06;c1 = [120 150 230]/255;c2 = ([120 150 230]+0)/383;c3 = ([120 150 230]+128)/383;patch([0 1 1 0],[0 0 1 1],c1);patch([0 1 1 1-e 1-e 0+e],[0 0 1 1-e 0+e 0+e],c2);patch([0 0 1 1-e 0+e 0+e],[0 1 1 1-e 1-e 0+e],c3);plot([0 1 1 0 0],[0 0 1 1 0]);disp('Weights');
  "IW{1,1}(62,:)'" : Constant  Value=[-0.17042134725705959663599742270889692008495330810546875;1.0560137602958992175672392477281391620635986328125;0.63897153620610913637989369817660190165042877197265625;-0.65316188570588862294385990026057697832584381103515625;0.6317779224873574239751405912102200090885162353515625;-1.987904298449198581266728069749660789966583251953125;1.018946150341101475333971393411047756671905517578125]
      mask Display: e = 0.06;c1 = [120 150 230]/255;c2 = ([120 150 230]+0)/383;c3 = ([120 150 230]+128)/383;patch([0 1 1 0],[0 0 1 1],c1);patch([0 1 1 1-e 1-e 0+e],[0 0 1 1-e 0+e 0+e],c2);patch([0 0 1 1-e 0+e 0+e],[0 1 1 1-e 1-e 0+e],c3);plot([0 1 1 0 0],[0 0 1 1 0]);disp('Weights');
  "IW{1,1}(63,:)'" : Constant  Value=[-0.7910782245755407782183965537115000188350677490234375;0.738394424065875742968501072027720510959625244140625;0.39570458294022958778413112668204121291637420654296875;0.6948746501498452854406195910996757447719573974609375;0.6104256817513853405898771598003804683685302734375;1.8595814179841354540911879666964523494243621826171875;-1.062203346308225437866212814697064459323883056640625]
      mask Display: e = 0.06;c1 = [120 150 230]/255;c2 = ([120 150 230]+0)/383;c3 = ([120 150 230]+128)/383;patch([0 1 1 0],[0 0 1 1],c1);patch([0 1 1 1-e 1-e 0+e],[0 0 1 1-e 0+e 0+e],c2);patch([0 0 1 1-e 0+e 0+e],[0 1 1 1-e 1-e 0+e],c3);plot([0 1 1 0 0],[0 0 1 1 0]);disp('Weights');
  "IW{1,1}(64,:)'" : Constant  Value=[-1.207787224619776278444760464481078088283538818359375;1.0769569352047139165762246193480677902698516845703125;-1.3487434395624877669916941158589906990528106689453125;-0.9914292861352447250311570314806886017322540283203125;0.96162714418659422932478264556266367435455322265625;0.09192610714386821590959897321226890198886394500732421875;0.366031925305908389933762236978509463369846343994140625]
      mask Display: e = 0.06;c1 = [120 150 230]/255;c2 = ([120 150 230]+0)/383;c3 = ([120 150 230]+128)/383;patch([0 1 1 0],[0 0 1 1],c1);patch([0 1 1 1-e 1-e 0+e],[0 0 1 1-e 0+e 0+e],c2);patch([0 0 1 1-e 0+e 0+e],[0 1 1 1-e 1-e 0+e],c3);plot([0 1 1 0 0],[0 0 1 1 0]);disp('Weights');
  "IW{1,1}(7,:)'" : Constant  Value=[-0.11676038563379816104248476449356530793011188507080078125;1.261018417038072936264825329999439418315887451171875;0.61587380171800443218188547689351253211498260498046875;-1.3041433149450203377028856266406364738941192626953125;-1.0161732097028159937934788104030303657054901123046875;1.043136290417156164522793915239162743091583251953125;0.9211484263394267291147343712509609758853912353515625]
      mask Display: e = 0.06;c1 = [120 150 230]/255;c2 = ([120 150 230]+0)/383;c3 = ([120 150 230]+128)/383;patch([0 1 1 0],[0 0 1 1],c1);patch([0 1 1 1-e 1-e 0+e],[0 0 1 1-e 0+e 0+e],c2);patch([0 0 1 1-e 0+e 0+e],[0 1 1 1-e 1-e 0+e],c3);plot([0 1 1 0 0],[0 0 1 1 0]);disp('Weights');
  "IW{1,1}(8,:)'" : Constant  Value=[-1.1978067316522420515667590734665282070636749267578125;-0.1523005135221014716417897716382867656648159027099609375;0.3939518184864965189007079970906488597393035888671875;1.28598090633823591844020484131760895252227783203125;0.5031145563842418511057985597290098667144775390625;-2.156899122677105484768844689824618399143218994140625;-0.90123718807132136010551448634942062199115753173828125]
      mask Display: e = 0.06;c1 = [120 150 230]/255;c2 = ([120 150 230]+0)/383;c3 = ([120 150 230]+128)/383;patch([0 1 1 0],[0 0 1 1],c1);patch([0 1 1 1-e 1-e 0+e],[0 0 1 1-e 0+e 0+e],c2);patch([0 0 1 1-e 0+e 0+e],[0 1 1 1-e 1-e 0+e],c3);plot([0 1 1 0 0],[0 0 1 1 0]);disp('Weights');
  "IW{1,1}(9,:)'" : Constant  Value=[-3.7146126207903051863468135707080364227294921875;1.8050017234581112735014585268800146877765655517578125;0.5600911336280807173437779056257568299770355224609375;-0.485969311568317241523118354962207376956939697265625;0.380280107309155679384815584853640757501125335693359375;2.553903138663950134201741093420423567295074462890625;1.7744120992394882829756852515856735408306121826171875]
      mask Display: e = 0.06;c1 = [120 150 230]/255;c2 = ([120 150 230]+0)/383;c3 = ([120 150 230]+128)/383;patch([0 1 1 0],[0 0 1 1],c1);patch([0 1 1 1-e 1-e 0+e],[0 0 1 1-e 0+e 0+e],c2);patch([0 0 1 1-e 0+e 0+e],[0 1 1 1-e 1-e 0+e],c3);plot([0 1 1 0 0],[0 0 1 1 0]);disp('Weights');
  Mux : Mux  Inputs=64
      mask Display: e = 0.06;c1 = [120 150 230]/255;c2 = ([120 150 230]+0)/383;c3 = ([120 150 230]+128)/383;patch([0 1 1 0],[0 0 1 1],c1);patch([0 1 1 1-e 1-e 0+e],[0 0 1 1-e 0+e 0+e],c2);patch([0 0 1 1-e 0+e 0+e],[0 1 1 1-e 1-e 0+e],c3);plot([0 1 1 0 0],[0 0 1 1 0]);disp('Mux');
  dotprod{1..64} (64 alike) : neural/Weight Functions/dotprod
  "iz{1,1}" : Outport
      mask Display: e = 0.06;c1 = [120 230 180]/255;c2 = ([120 230 180]+0)/(256+128);c3 = ([120 230 180]+128)/(256+128);patch([0 1 1 0],[0 0 1 1],c1);patch([0 1 1 1-e 1-e 0+e],[0 0 1 1-e 0+e 0+e],c2);patch([0 0 1 1-e 0+e 0+e],[0 1 1 1-e 1-e 0+e],c3);plot([0 1 1 0 0],[0 0 1 1 0]);
  wires:
  "IW{1,1}(1,:)'"/1 -> dotprod1/1
  "pd{1,1}"/1 -> dotprod1/2, dotprod2/2, dotprod3/2, dotprod4/2, dotprod5/2, dotprod6/2, dotprod7/2, dotprod8/2, dotprod9/2, dotprod10/2, dotprod11/2, dotprod12/2, dotprod13/2, dotprod14/2, dotprod15/2, dotprod16/2, dotprod17/2, dotprod18/2, dotprod19/2, dotprod20/2, dotprod21/2, dotprod22/2, dotprod23/2, dotprod24/2, dotprod25/2, dotprod26/2, dotprod27/2, dotprod28/2, dotprod29/2, dotprod30/2, dotprod31/2, dotprod32/2, dotprod33/2, dotprod34/2, dotprod35/2, dotprod36/2, dotprod37/2, dotprod38/2, dotprod39/2, dotprod40/2, dotprod41/2, dotprod42/2, dotprod43/2, dotprod44/2, dotprod45/2, dotprod46/2, dotprod47/2, dotprod48/2, dotprod49/2, dotprod50/2, dotprod51/2, dotprod52/2, dotprod53/2, dotprod54/2, dotprod55/2, dotprod56/2, dotprod57/2, dotprod58/2, dotprod59/2, dotprod60/2, dotprod61/2, dotprod62/2, dotprod63/2, dotprod64/2
  dotprod1/1 -> Mux/1
  "IW{1,1}(2,:)'"/1 -> dotprod2/1
  dotprod2/1 -> Mux/2
  "IW{1,1}(3,:)'"/1 -> dotprod3/1
  dotprod3/1 -> Mux/3
  "IW{1,1}(4,:)'"/1 -> dotprod4/1
  dotprod4/1 -> Mux/4
  "IW{1,1}(5,:)'"/1 -> dotprod5/1
  dotprod5/1 -> Mux/5
  "IW{1,1}(6,:)'"/1 -> dotprod6/1
  dotprod6/1 -> Mux/6
  "IW{1,1}(7,:)'"/1 -> dotprod7/1
  dotprod7/1 -> Mux/7
  "IW{1,1}(8,:)'"/1 -> dotprod8/1
  dotprod8/1 -> Mux/8
  "IW{1,1}(9,:)'"/1 -> dotprod9/1
  dotprod9/1 -> Mux/9
  "IW{1,1}(10,:)'"/1 -> dotprod10/1
  dotprod10/1 -> Mux/10
  "IW{1,1}(11,:)'"/1 -> dotprod11/1
  dotprod11/1 -> Mux/11
  "IW{1,1}(12,:)'"/1 -> dotprod12/1
  dotprod12/1 -> Mux/12
  "IW{1,1}(13,:)'"/1 -> dotprod13/1
  dotprod13/1 -> Mux/13
  "IW{1,1}(14,:)'"/1 -> dotprod14/1
  dotprod14/1 -> Mux/14
  "IW{1,1}(15,:)'"/1 -> dotprod15/1
  dotprod15/1 -> Mux/15
  "IW{1,1}(16,:)'"/1 -> dotprod16/1
  dotprod16/1 -> Mux/16
  "IW{1,1}(17,:)'"/1 -> dotprod17/1
  dotprod17/1 -> Mux/17
  "IW{1,1}(18,:)'"/1 -> dotprod18/1
  dotprod18/1 -> Mux/18
  "IW{1,1}(19,:)'"/1 -> dotprod19/1
  dotprod19/1 -> Mux/19
  "IW{1,1}(20,:)'"/1 -> dotprod20/1
  dotprod20/1 -> Mux/20
  "IW{1,1}(21,:)'"/1 -> dotprod21/1
  dotprod21/1 -> Mux/21
  "IW{1,1}(22,:)'"/1 -> dotprod22/1
  dotprod22/1 -> Mux/22
  "IW{1,1}(23,:)'"/1 -> dotprod23/1
  dotprod23/1 -> Mux/23
  "IW{1,1}(24,:)'"/1 -> dotprod24/1
  dotprod24/1 -> Mux/24
  "IW{1,1}(25,:)'"/1 -> dotprod25/1
  dotprod25/1 -> Mux/25
  "IW{1,1}(26,:)'"/1 -> dotprod26/1
  dotprod26/1 -> Mux/26
  "IW{1,1}(27,:)'"/1 -> dotprod27/1
  dotprod27/1 -> Mux/27
  "IW{1,1}(28,:)'"/1 -> dotprod28/1
  dotprod28/1 -> Mux/28
  "IW{1,1}(29,:)'"/1 -> dotprod29/1
  dotprod29/1 -> Mux/29
  "IW{1,1}(30,:)'"/1 -> dotprod30/1
  dotprod30/1 -> Mux/30
  "IW{1,1}(31,:)'"/1 -> dotprod31/1
  dotprod31/1 -> Mux/31
  "IW{1,1}(32,:)'"/1 -> dotprod32/1
  dotprod32/1 -> Mux/32
  "IW{1,1}(33,:)'"/1 -> dotprod33/1
  dotprod33/1 -> Mux/33
  "IW{1,1}(34,:)'"/1 -> dotprod34/1
  dotprod34/1 -> Mux/34
  "IW{1,1}(35,:)'"/1 -> dotprod35/1
  dotprod35/1 -> Mux/35
  "IW{1,1}(36,:)'"/1 -> dotprod36/1
  dotprod36/1 -> Mux/36
  "IW{1,1}(37,:)'"/1 -> dotprod37/1
  dotprod37/1 -> Mux/37
  "IW{1,1}(38,:)'"/1 -> dotprod38/1
  dotprod38/1 -> Mux/38
  "IW{1,1}(39,:)'"/1 -> dotprod39/1
  dotprod39/1 -> Mux/39
  "IW{1,1}(40,:)'"/1 -> dotprod40/1
  dotprod40/1 -> Mux/40
  "IW{1,1}(41,:)'"/1 -> dotprod41/1
  dotprod41/1 -> Mux/41
  "IW{1,1}(42,:)'"/1 -> dotprod42/1
  dotprod42/1 -> Mux/42
  "IW{1,1}(43,:)'"/1 -> dotprod43/1
  dotprod43/1 -> Mux/43
  "IW{1,1}(44,:)'"/1 -> dotprod44/1
  dotprod44/1 -> Mux/44
  "IW{1,1}(45,:)'"/1 -> dotprod45/1
  dotprod45/1 -> Mux/45
  "IW{1,1}(46,:)'"/1 -> dotprod46/1
  dotprod46/1 -> Mux/46
  "IW{1,1}(47,:)'"/1 -> dotprod47/1
  dotprod47/1 -> Mux/47
  "IW{1,1}(48,:)'"/1 -> dotprod48/1
  dotprod48/1 -> Mux/48
  "IW{1,1}(49,:)'"/1 -> dotprod49/1
  dotprod49/1 -> Mux/49
  "IW{1,1}(50,:)'"/1 -> dotprod50/1
  dotprod50/1 -> Mux/50
  "IW{1,1}(51,:)'"/1 -> dotprod51/1
  dotprod51/1 -> Mux/51
  "IW{1,1}(52,:)'"/1 -> dotprod52/1
  dotprod52/1 -> Mux/52
  "IW{1,1}(53,:)'"/1 -> dotprod53/1
  dotprod53/1 -> Mux/53
  "IW{1,1}(54,:)'"/1 -> dotprod54/1
  dotprod54/1 -> Mux/54
  "IW{1,1}(55,:)'"/1 -> dotprod55/1
  dotprod55/1 -> Mux/55
  "IW{1,1}(56,:)'"/1 -> dotprod56/1
  dotprod56/1 -> Mux/56
  "IW{1,1}(57,:)'"/1 -> dotprod57/1
  dotprod57/1 -> Mux/57
  "IW{1,1}(58,:)'"/1 -> dotprod58/1
  dotprod58/1 -> Mux/58
  "IW{1,1}(59,:)'"/1 -> dotprod59/1
  dotprod59/1 -> Mux/59
  "IW{1,1}(60,:)'"/1 -> dotprod60/1
  dotprod60/1 -> Mux/60
  "IW{1,1}(61,:)'"/1 -> dotprod61/1
  dotprod61/1 -> Mux/61
  "IW{1,1}(62,:)'"/1 -> dotprod62/1
  dotprod62/1 -> Mux/62
  "IW{1,1}(63,:)'"/1 -> dotprod63/1
  dotprod63/1 -> Mux/63
  "IW{1,1}(64,:)'"/1 -> dotprod64/1
  dotprod64/1 -> Mux/64
  Mux/1 -> "iz{1,1}"/1
